simulink model "projectcircuit"  (Simulink 8.3)
settings: Solver=ode23tb  StartTime=0.0  StopTime=0.1  MaxStep=1e-6  RelTol=1e-3
libraries: powerlib x16, simulink x8
settings Model: Creator=nittu  LastModifiedBy=nittu
settings DataIOCC: SignalLoggingSaveFormat=Dataset
settings DebuggingCC: UnderspecifiedInitializationDetection=Simplified  StateNameClashWarn=none
settings GRTTargetCC: CombineOutputUpdateFcns=on  GRTInterface=off

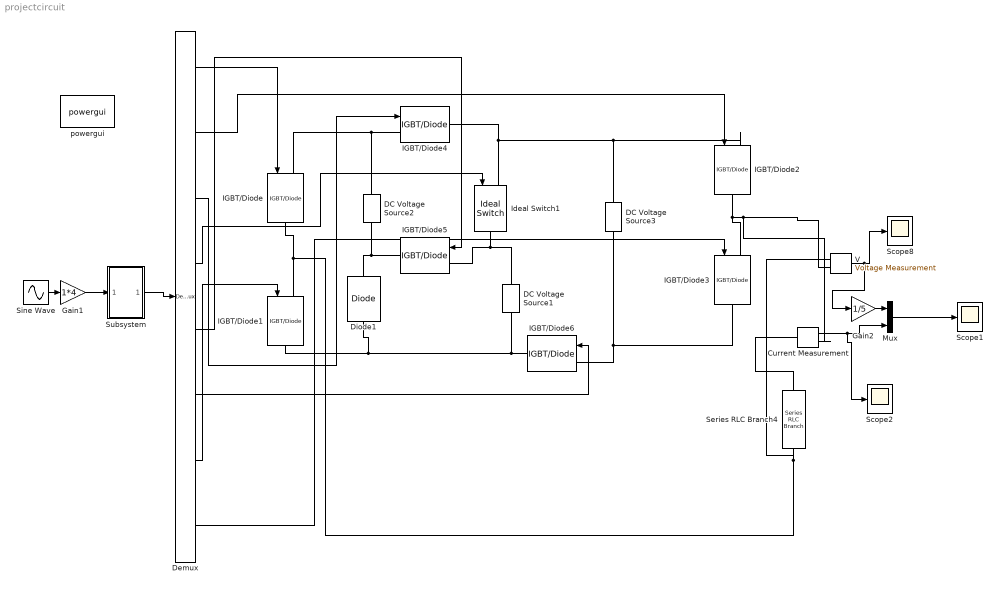
== system projectcircuit ==
  Current Measurement : powerlib/Measurements/Current Measurement  PhasorSimulation=off  OutputType=Complex  PSBequivalent=0
  DC Voltage Source1 : powerlib/Electrical Sources/DC Voltage Source  Amplitude=100  Measurements=None
  DC Voltage Source2 : powerlib/Electrical Sources/DC Voltage Source  Amplitude=100  Measurements=None
  DC Voltage Source3 : powerlib/Electrical Sources/DC Voltage Source  Amplitude=50  Measurements=None
  Demux : Demux  Outputs=8
  Diode1 : powerlib/Power Electronics/Diode  Ron=0.001  Lon=0  Vf=0.8  IC=0  UseSnubber=off  Rs=500  Cs=250e-9  Measurements=off
  Gain1 : Gain  Gain=1*4
  Gain2 : Gain  Gain=1/5
  IGBT/Diode{,1..6} (7 alike) : powerlib/Power Electronics/IGBT//Diode  Ron=1e-3  Rs=1e5  Cs=inf  Measurements=off
  Ideal Switch1 : powerlib/Power Electronics/Ideal Switch  Ron=0.001  Lon=0  IC=0  Rs=1e5  Cs=inf  Measurements=off
  Mux : Mux  Inputs=2
  Scope1 : Scope
      settings: TimeRange=0.1  YMax=4  SaveName=ScopeData4  SampleTime=10e-6
  Scope2 : Scope
      settings: TimeRange=0.1  YMax=4  SaveName=opvc1  SampleTime=10e-6
  Scope8 : Scope
      settings: TimeRange=0.1  YMin=-150  YMax=150  SaveName=opvc8  SampleTime=10e-6
  Series RLC Branch4 : powerlib/Elements/Series RLC Branch  LConnTagsString=__new0  RConnTagsString=__new0  BranchType=RL  Resistance=150  Inductance=50e-3  SetiL0=off  InitialCurrent=0  Capacitance=inf  Setx0=off  InitialVoltage=0  Measurements=None
  Sine Wave : Sin  Frequency=2*50*3.14  SampleTime=0
  Subsystem : Subsystem
  V : powerlib/Measurements/Voltage Measurement  PhasorSimulation=off  OutputType=Complex  PSBequivalent=0
  powergui : powerlib/powergui  Priority=1  SimulationMode=Continuous  SolverType=Tustin  SampleTime=50e-6  frequency=60  SPID=off  DisableSnubberDevices=off  DisableRonSwitches=off  DisableVfSwitches=off  SwTol=0  Interpol=off  DisplayEquations=off  Ts=0  methode=off  frequencyindice=0  Pbase=100e6  ErrMax=1e-4  Iterations=50  UnitsV=kV  UnitsW=MW  FunctionMessages=off  echomessages=off  HookPort=off  EnableUseOfTLC=off  x0status=blocks  RestoreLinks=warning  ResistiveCurrentMeasurement=off  Frange=[0:2:500]  Ylog=off  Xlog=on  ShowGrid=off  save=off  variable=ZData  structure=opvc8  ZoomFFT=on  StartTime=0.0  cycles=5  DisplayStyle=2  fundamental=50  FreqAxis=on  MaxFrequency=2050  frequencyindicesteady=1  RmsSteady=1  display=off
  wires:
  V/1 -> Gain2/1, Scope8/1
  Sine Wave/1 -> Gain1/1
  Gain1/1 -> Subsystem/1(In1)
  Subsystem/1(Out1) -> Demux/1
  Demux/1 -> IGBT/Diode/1
  Demux/2 -> IGBT/Diode2/1
  Demux/3 -> IGBT/Diode4/1
  Demux/4 -> Ideal Switch1/1
  Demux/5 -> IGBT/Diode5/1
  Demux/6 -> IGBT/Diode6/1
  Demux/7 -> IGBT/Diode1/1
  Demux/8 -> IGBT/Diode3/1
  Current Measurement/1 -> Scope2/1, Mux/2
  Mux/1 -> Scope1/1
  Gain2/1 -> Mux/1
  connections:
  DC Voltage Source1/LConn1 -- IGBT/Diode6/RConn1 -- IGBT/Diode1/RConn1 -- Diode1/LConn1
  V/LConn1 -- Series RLC Branch4/RConn1 -- IGBT/Diode1/LConn1 -- IGBT/Diode/RConn1
  IGBT/Diode4/LConn1 -- IGBT/Diode/LConn1 -- DC Voltage Source2/RConn1
  DC Voltage Source3/RConn1 -- IGBT/Diode2/LConn1 -- Ideal Switch1/LConn1 -- IGBT/Diode4/RConn1
  Ideal Switch1/RConn1 -- IGBT/Diode5/LConn1 -- DC Voltage Source1/RConn1
  IGBT/Diode3/RConn1 -- DC Voltage Source3/LConn1 -- IGBT/Diode6/LConn1
  Current Measurement/RConn1 -- V/LConn2 -- IGBT/Diode3/LConn1 -- IGBT/Diode2/RConn1
  Current Measurement/LConn1 -- Series RLC Branch4/LConn1
  IGBT/Diode5/RConn1 -- DC Voltage Source2/LConn1 -- Diode1/RConn1

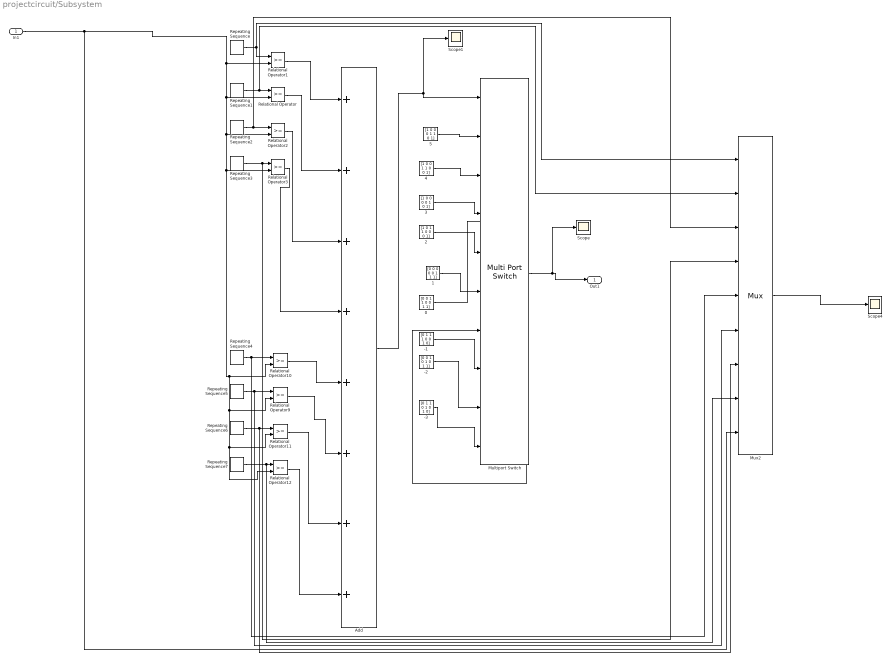
== system projectcircuit/Subsystem ==
  In1 : Inport
  -1 : Constant  Value="[0\t1\t1\t1\t0\t0\t1\t0]"
  -2 : Constant  Value="[0\t0\t1\t0\t1\t0\t1\t1]"
  -3 : Constant  Value="[0\t1\t1\t0\t1\t0\t1\t0]"
  0 : Constant  Value="[0\t0\t1\t1\t0\t0\t1\t1]"
  1 : Constant  Value="[0\t0\t0\t0\t0\t1\t1\t1]"
  2 : Constant  Value="[1\t0\t1\t1\t0\t0\t0\t1]"
  3 : Constant  Value="[1\t0\t0\t0\t0\t1\t0\t1]"
  4 : Constant  Value="[1\t0\t0\t1\t1\t0\t0\t1]"
  5 : Constant  Value="[1\t0\t0\t0\t1\t1\t0\t1]"
  Add : Sum  Inputs=++++++++
  Multiport Switch : MultiPortSwitch  DataPortOrder=Specify indices  Inputs=19  DataPortIndices={0,1,2,3,4,5,6,7,8}  DiagnosticForDefault=None
  Mux2 : Mux  Inputs=9
  Relational Operator{,1..3,9..12} (8 alike) : RelationalOperator  OutDataTypeStr=boolean
  Repeating Sequence : simulink/Sources/Repeating Sequence  rep_seq_t=[0 0.5/1000 1/2000]  rep_seq_y=[0 1 0]
  Repeating Sequence1 : simulink/Sources/Repeating Sequence  rep_seq_t=[0 0.5/2000 1/2000]  rep_seq_y=[2 1 2]
  Repeating Sequence2 : simulink/Sources/Repeating Sequence  rep_seq_t=[0 0.5/1000 1/2000]  rep_seq_y=[2 3 2]
  Repeating Sequence3 : simulink/Sources/Repeating Sequence  rep_seq_t=[0 0.5/2000 1/2000]  rep_seq_y=[4 3 4]
  Repeating Sequence4 : simulink/Sources/Repeating Sequence  rep_seq_t=[0 0.5/1000 1/2000]  rep_seq_y=[0 -1 0]
  Repeating Sequence5 : simulink/Sources/Repeating Sequence  rep_seq_t=[0 0.5/2000 1/2000]  rep_seq_y=[-2 -1 -2]
  Repeating Sequence6 : simulink/Sources/Repeating Sequence  rep_seq_t=[0 0.5/1000 1/2000]  rep_seq_y=[-2 -3 -2]
  Repeating Sequence7 : simulink/Sources/Repeating Sequence  rep_seq_t=[0 0.5/2000 1/2000]  rep_seq_y=[-4 -3 -4]
  Scope : Scope
      settings: SaveName=output
  Scope1 : Scope
      settings: TimeRange=0.008  YMax=4  SaveName=op  SampleTime=10e-6
  Scope4 : Scope
      settings: TimeRange=0.008  YMax=4  SaveName=opvc13  SampleTime=10e-6
  Out1 : Outport
  wires:
  Repeating Sequence/1 -> Relational Operator1/1, Mux2/1
  Repeating Sequence1/1 -> Mux2/2, Relational Operator/1
  Repeating Sequence2/1 -> Mux2/3, Relational Operator2/1
  Repeating Sequence3/1 -> Mux2/4, Relational Operator3/1
  Relational Operator3/1 -> Add/4
  Relational Operator2/1 -> Add/3
  Relational Operator/1 -> Add/2
  Relational Operator1/1 -> Add/1
  Add/1 -> Scope1/1, Multiport Switch/1
  Multiport Switch/1 -> Scope/1, Out1/1
  Repeating Sequence4/1 -> Mux2/5, Relational Operator10/1
  Repeating Sequence5/1 -> Mux2/6, Relational Operator9/1
  Repeating Sequence6/1 -> Mux2/7, Relational Operator11/1
  Repeating Sequence7/1 -> Mux2/8, Relational Operator12/1
  Relational Operator12/1 -> Add/8
  Relational Operator11/1 -> Add/7
  Relational Operator9/1 -> Add/6
  Relational Operator10/1 -> Add/5
  5/1 -> Multiport Switch/2
  4/1 -> Multiport Switch/3
  3/1 -> Multiport Switch/4
  2/1 -> Multiport Switch/5
  1/1 -> Multiport Switch/6
  0/1 -> Multiport Switch/7
  -1/1 -> Multiport Switch/8
  -2/1 -> Multiport Switch/9
  -3/1 -> Multiport Switch/10
  Mux2/1 -> Scope4/1
  In1/1 -> Mux2/9, Relational Operator1/2, Relational Operator12/2, Relational Operator11/2, Relational Operator9/2, Relational Operator10/2, Relational Operator3/2, Relational Operator2/2, Relational Operator/2
